simulink model "openMHA_test_gaintable"  (R2020a)
settings: Solver=VariableStepAuto  StartTime=0.0  StopTime=stop_time  RelTol=1e-3
InitFcn:
  | test_gaintable_init
StopFcn:
  | test_gaintable_stop
values from neighbouring files (symbols this model uses):
  dp_gt = gt'    [test_FFT_to_gain_init.m]    (also in test_ar_filter_gaintable_init.m; test_db_ar_gaintable_init.m; test_db_lookup_gain_fpga_init.m; test_db_lookup_init.m)
  table_length = length(gtdata)    [calculate_gaintable.m]    (also in test_FFT_to_gain_init.m; test_ar_filter_gaintable_init.m; test_db_ar_gaintable_init.m; test_db_lookup_gain_fpga_init.m)
libraries: dspsrcs4 x7, FPGA_Open_Speech_Tools x1
settings Model: Creator=t96f346  LastModifiedBy=t96f346

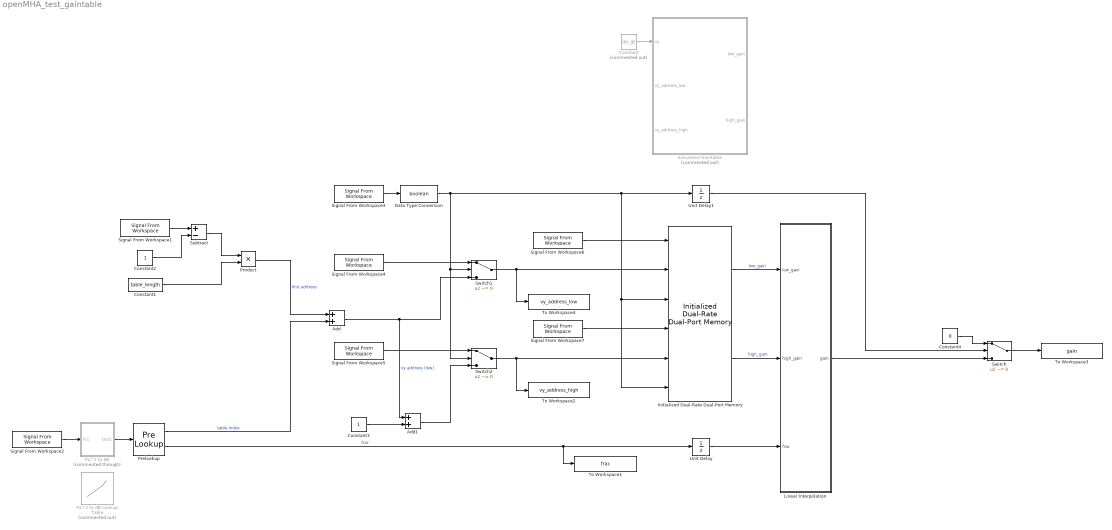
== system openMHA_test_gaintable ==
  Add : Sum  OutDataTypeStr=uint8
  Add1 : Sum  OutDataTypeStr=uint8
  Constant : Constant  Commented=on  Value=dp_gt  SampleTime=-1
  Constant1 : Constant  Value=table_length  OutDataTypeStr=uint8  SampleTime=-1
  Constant2 : Constant  OutDataTypeStr=uint8  SampleTime=-1
  Constant3 : Constant  OutDataTypeStr=uint8  SampleTime=-1
  Constant4 : Constant  Value=0  OutDataTypeStr=double  SampleTime=-1
  Data Type Conversion : DataTypeConversion  OutDataTypeStr=boolean
  Initialized Dual-Rate Dual-Port Memory : FPGA_Open_Speech_Tools/Initialized Dual-Rate Dual-Port Memory  ram_size=RAM_size  Table_Init=vy
      settings: SourceProductName=FPGA Open Speech Tools
  Linear Interpolation : Subsystem
  Pa^2 to dB : Subsystem  Commented=through
  Pa^2 to dB Lookup Table : Lookup_n-D  Commented=on  NumberOfTableDimensions=1  LookupTableObject=''  BreakpointsForDimension1=[-5:5]  BreakpointsForDimension1FirstPoint=10  BreakpointsForDimension2FirstPoint=10  BreakpointsForDimension1Spacing=12  BreakpointsForDimension2Spacing=12  IndexSearchMethod=Evenly spaced points  Table=tanh([-5:5])  InterpMethod=Flat  DiagnosticForOutOfRangeInput=Error  InternalRulePriority=Speed  RndMeth=Simplest  InputSameDT=on
  Prelookup : PreLookup  BreakpointsData=input_levels_db  IndexSearchMethod=Evenly spaced points  UseLastBreakpoint=on  DiagnosticForOutOfRangeInput=Error  IndexDataTypeStr=uint8
  Product : Product  OutDataTypeStr=Inherit: Same as first input
  Signal From Workspace1 : dspsrcs4/Signal From Workspace  X=band_num  Ts=1  nsamps=1  OutputAfterFinalValue=Setting to zero  ignoreOrWarnInputAndFrameLengths=off  OutputFrames=off
  Signal From Workspace2 : dspsrcs4/Signal From Workspace  X=level_in_filtered  Ts=1  nsamps=1  OutputAfterFinalValue=Setting to zero  ignoreOrWarnInputAndFrameLengths=off  OutputFrames=off
  Signal From Workspace3 : dspsrcs4/Signal From Workspace  X=write_en  Ts=1  nsamps=1  OutputAfterFinalValue=Setting to zero  ignoreOrWarnInputAndFrameLengths=off  OutputFrames=off
  Signal From Workspace4 : dspsrcs4/Signal From Workspace  X=write_addrA  Ts=1  nsamps=1  OutputAfterFinalValue=Setting to zero  ignoreOrWarnInputAndFrameLengths=off  OutputFrames=off
  Signal From Workspace5 : dspsrcs4/Signal From Workspace  X=write_addrB  Ts=1  nsamps=1  OutputAfterFinalValue=Setting to zero  ignoreOrWarnInputAndFrameLengths=off  OutputFrames=off
  Signal From Workspace6 : dspsrcs4/Signal From Workspace  X=write_dataA  Ts=1  nsamps=1  OutputAfterFinalValue=Setting to zero  ignoreOrWarnInputAndFrameLengths=off  OutputFrames=off
  Signal From Workspace7 : dspsrcs4/Signal From Workspace  X=write_dataB  Ts=1  nsamps=1  OutputAfterFinalValue=Setting to zero  ignoreOrWarnInputAndFrameLengths=off  OutputFrames=off
  Simulated Gaintable : MATLAB Function  Commented=on  TreatAsAtomicUnit=on
  Subtract : Sum  Inputs=+-
  Switch : Switch  Criteria=u2 ~= 0  OutDataTypeStr=double
  Switch1 : Switch  Criteria=u2 ~= 0  OutDataTypeStr=uint8
  Switch2 : Switch  Criteria=u2 ~= 0  OutDataTypeStr=uint8
  To Workspace1 : ToWorkspace  VariableName=frac  SampleTime=-1
      settings: Save2DSignal=2-D array (concatenate along first dimension)
  To Workspace2 : ToWorkspace  VariableName=vy_address_high  SampleTime=-1
      settings: Save2DSignal=2-D array (concatenate along first dimension)
  To Workspace3 : ToWorkspace  VariableName=gain  SampleTime=-1
      settings: Save2DSignal=2-D array (concatenate along first dimension)
  To Workspace4 : ToWorkspace  VariableName=vy_address_low  SampleTime=-1
      settings: Save2DSignal=2-D array (concatenate along first dimension)
  Unit Delay : UnitDelay  SampleTime=-1  HasFrameUpgradeWarning=on
  Unit Delay1 : UnitDelay  InitialCondition=1  SampleTime=-1  HasFrameUpgradeWarning=on
  wires:
  Signal From Workspace2/1 -> Pa^2 to dB/1(In1)
  Signal From Workspace1/1 -> Subtract/1
  Constant2/1 -> Subtract/2
  Subtract/1 -> Product/1
  Constant1/1 -> Product/2
  Product/1 -> Add/1  "first address"
  Prelookup/1 -> Add/2  "table index"
  Add/1 -> Switch1/3, Add1/1  "vy address (low)"
  Prelookup/2 -> To Workspace1/1, Unit Delay/1  "frac"
  Constant3/1 -> Add1/2
  Add1/1 -> Switch2/3
  Pa^2 to dB/1(Out1) -> Prelookup/1
  Initialized Dual-Rate Dual-Port Memory/1 -> Linear Interpolation/1(low_gain)  "low_gain"
  Initialized Dual-Rate Dual-Port Memory/2 -> Linear Interpolation/2(high_gain)  "high_gain"
  Linear Interpolation/1(gain) -> Switch/3
  Constant/1 -> Simulated Gaintable/1(vy)
  Unit Delay/1 -> Linear Interpolation/3(frac)
  Signal From Workspace3/1 -> Data Type Conversion/1
  Data Type Conversion/1 -> Initialized Dual-Rate Dual-Port Memory/3, Initialized Dual-Rate Dual-Port Memory/6, Unit Delay1/1, Switch1/2, Switch2/2
  Unit Delay1/1 -> Switch/2
  Constant4/1 -> Switch/1
  Switch/1 -> To Workspace3/1
  Signal From Workspace4/1 -> Switch1/1
  Signal From Workspace5/1 -> Switch2/1
  Switch2/1 -> Initialized Dual-Rate Dual-Port Memory/5, To Workspace2/1
  Signal From Workspace7/1 -> Initialized Dual-Rate Dual-Port Memory/4
  Signal From Workspace6/1 -> Initialized Dual-Rate Dual-Port Memory/1
  Switch1/1 -> Initialized Dual-Rate Dual-Port Memory/2, To Workspace4/1

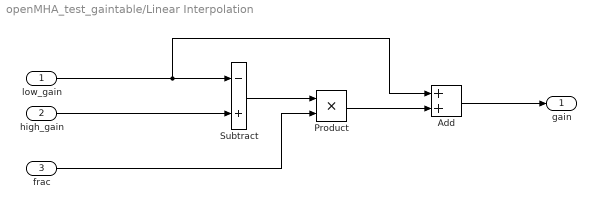
== system openMHA_test_gaintable/Linear Interpolation ==
  low_gain : Inport
  high_gain : Inport  Port=2
  frac : Inport  Port=3
  Add : Sum
  Product : Product
  Subtract : Sum  Inputs=-+
  gain : Outport
  wires:
  high_gain/1 -> Subtract/2
  low_gain/1 -> Add/1, Subtract/1
  Subtract/1 -> Product/1
  frac/1 -> Product/2
  Product/1 -> Add/2
  Add/1 -> gain/1

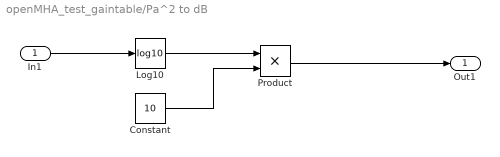
== system openMHA_test_gaintable/Pa^2 to dB ==
  In1 : Inport
  Constant : Constant  Value=10  SampleTime=-1
  Log10 : Math  Operator=log10  SaturateOnIntegerOverflow=on
  Product : Product
  Out1 : Outport
  wires:
  In1/1 -> Log10/1
  Product/1 -> Out1/1
  Log10/1 -> Product/1
  Constant/1 -> Product/2

== matlab function openMHA_test_gaintable/Simulated Gaintable ==
  data: vy input; low_gain output; vy_address_low input; vy_address_high input; high_gain output
function [low_gain, high_gain] = gaintable(vy, vy_address_low, vy_address_high)

% Simulates a Dual Rate Dual Port Gain Table by taking in the gain table
% values along with the two calculated addresses that contain the
% appropriate gain values for the band in question.

low_gain = vy(vy_address_low + 1);
high_gain = vy(vy_address_high + 1);
